simulink model "eulerPropagate"  (R2023b)
settings: Solver=VariableStepAuto  StartTime=0.0  StopTime=Tfinal  MaxStep=3  RelTol=1e-3
model workspace: external: MATLAB File plantConstants.m (data not in the file)
values from neighbouring files (symbols this model uses):
  A_ptob = [0.00452111179393  0.994865050863  -0.101109297888; -0.99864921572  -0.000741813086313  -0.051953764597; -0.0517619888586  0.101207609816  0.993517848971]    [magConstants.mat]
undefined symbols (not defined in the file or in its folder): axesFlag, I_sim, Ir, om0, omr, r
settings Model: Creator=stanforduser  LastModifiedBy=kristopherriordan
settings DataIOCC: ExternalInput=[t,u]  SaveTime=off  ReturnWorkspaceOutputs=off  OutputSaveName=om

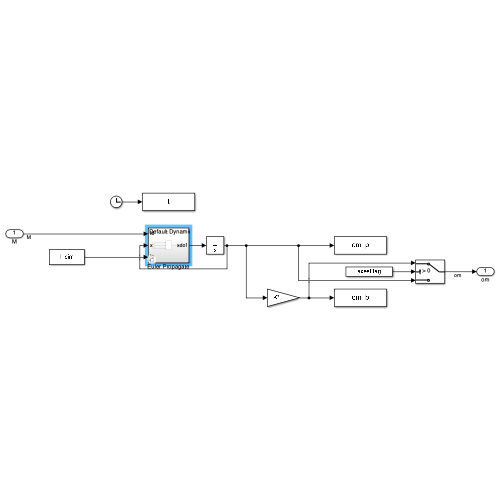
[thumbnail: Simulink's stored preview of the top-level diagram]
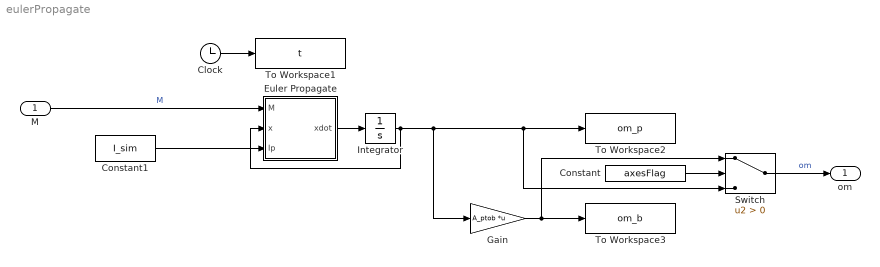
== system eulerPropagate ==
  M : Inport
  Clock : Clock
  Constant : Constant  Value=axesFlag
  Constant1 : Constant  Value=I_sim  VectorParams1D=off
  Euler Propagate : Subsystem  Variant=on  VariantControl=Euler Propagate
  Gain : Gain  Gain=A_ptob  Multiplication=Matrix(K*u)
  Integrator : Integrator  InitialCondition=om0
  Switch : Switch  Criteria=u2 > Threshold  SaturateOnIntegerOverflow=off  InputSameDT=off
  To Workspace1 : ToWorkspace  VariableName=t  SampleTime=-1
      settings: Save2DSignal=2-D array (concatenate along first dimension)
  To Workspace2 : ToWorkspace  VariableName=om_p  SampleTime=-1
      settings: Save2DSignal=2-D array (concatenate along first dimension)
  To Workspace3 : ToWorkspace  VariableName=om_b  SampleTime=-1
      settings: Save2DSignal=2-D array (concatenate along first dimension)
  om : Outport
  wires:
  Gain/1 -> To Workspace3/1, Switch/1
  Switch/1 -> om/1  "om"
  Integrator/1 -> To Workspace2/1, Switch/3, Gain/1, Euler Propagate/2(x)
  Constant/1 -> Switch/2
  Clock/1 -> To Workspace1/1
  M/1 -> Euler Propagate/1(M)  "M"
  Constant1/1 -> Euler Propagate/3(Ip)
  Euler Propagate/1(xdot) -> Integrator/1

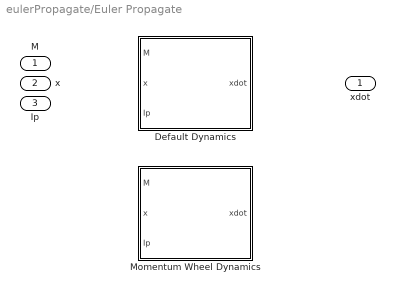
== system eulerPropagate/Euler Propagate ==
  M : Inport
  x : Inport  Port=2
  Ip : Inport  Port=3
  Default Dynamics : Subsystem  VariantControl="dynamicsType==\"default\""
  Momentum Wheel Dynamics : Subsystem  VariantControl="dynamicsType==\"wheel\""
  xdot : Outport

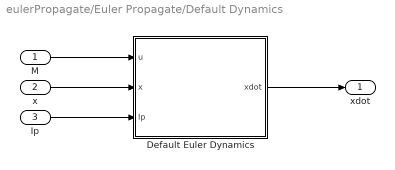
== system eulerPropagate/Euler Propagate/Default Dynamics ==
  M : Inport
  x : Inport  Port=2
  Ip : Inport  Port=3
  Default Euler Dynamics : MATLAB Function  TreatAsAtomicUnit=on
  xdot : Outport
  wires:
  Default Euler Dynamics/1(xdot) -> xdot/1
  Ip/1 -> Default Euler Dynamics/3(Ip)
  M/1 -> Default Euler Dynamics/1(u)
  x/1 -> Default Euler Dynamics/2(x)

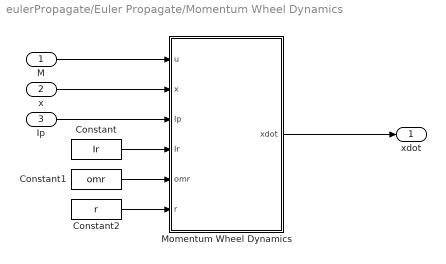
== system eulerPropagate/Euler Propagate/Momentum Wheel Dynamics ==
  M : Inport
  x : Inport  Port=2
  Ip : Inport  Port=3
  Constant : Constant  Value=Ir
  Constant1 : Constant  Value=omr
  Constant2 : Constant  Value=r  VectorParams1D=off
  Momentum Wheel Dynamics : MATLAB Function  TreatAsAtomicUnit=on
  xdot : Outport
  wires:
  Momentum Wheel Dynamics/1(xdot) -> xdot/1
  Ip/1 -> Momentum Wheel Dynamics/3(Ip)
  M/1 -> Momentum Wheel Dynamics/1(u)
  x/1 -> Momentum Wheel Dynamics/2(x)
  Constant/1 -> Momentum Wheel Dynamics/4(Ir)
  Constant1/1 -> Momentum Wheel Dynamics/5(omr)
  Constant2/1 -> Momentum Wheel Dynamics/6(r)

== matlab function eulerPropagate/Euler Propagate/Momentum Wheel Dynamics/Momentum Wheel Dynamics ==
  data: u input size=[3 1]; xdot output size=[3 1]; x input size=[3 1]; Ip input; Ir input; omr input; r input
function xdot = dualSpinDynamics(u,x,Ip,Ir,omr,r)

xdot = zeros(size(x));


Mx = u(1);
My = u(2);
Mz = u(3);

omx = x(1);
omy = x(2);
omz = x(3);

Ix = Ip(1,1);
Iy = Ip(2,2);
Iz = Ip(3,3);

rx = r(1);
ry = r(2);
rz = r(3);

wxdot = (1/Ix)*(Mx - ((Iz - Iy)*omy*omz + Ir*omr*(omy*rz - omz*ry)));
wydot = (1/Iy)*(My - ((Ix - Iz)*omz*omx + Ir*omr*(omz*rx - omx*rz)));
wzdot = (1/Iz)*(Mz - ((Iy - Ix)*omx*omy + Ir*omr*(omx*ry - omy*rx)));

xdot(1) = wxdot;
xdot(2) = wydot;
xdot(3) = wzdot;

end

== matlab function eulerPropagate/Euler Propagate/Default Dynamics/Default Euler Dynamics ==
  data: u input size=[3 1]; xdot output size=[3 1]; x input size=[3 1]; Ip input
function xdot = defaultDynamics(u,x,Ip)

xdot = zeros(size(x));


Mx = u(1);
My = u(2);
Mz = u(3);

omx = x(1);
omy = x(2);
omz = x(3);

Ix = Ip(1,1);
Iy = Ip(2,2);
Iz = Ip(3,3);

wxdot = (1/Ix)*(Mx - (Iz - Iy)*omy*omz);
wydot = (1/Iy)*(My - (Ix - Iz)*omz*omx);
wzdot = (1/Iz)*(Mz - (Iy - Ix)*omx*omy);

xdot(1) = wxdot;
xdot(2) = wydot;
xdot(3) = wzdot;

end
